simulink library "lib_dsphdlcontrol_v1"  (R2022a)
settings: Solver=ode45  StartTime=0.0  StopTime=10.0  RelTol=1e-3  EnableMultiTasking=on
undefined symbols (not defined in the file or in its folder): LIMIT, limit1, max1, min1, NumBits1, NumBits2, Slope1, Slope2, XMAX, XMIN
libraries: simulink x24, $bdroot x10, simulink_need_slupdate x5
settings Model: Creator=mbabst  LastModifiedBy=mbabst
settings SolverCC: AlgebraicLoopSolver=TrustRegion
settings DataIOCC: LimitDataPoints=on
settings OptimizationCC: LifeSpan=inf
settings DebuggingCC: UnconnectedInputMsg=warning  UnconnectedOutputMsg=warning  UnconnectedLineMsg=warning  AllowSymbolicDim=off  SFUnexpectedBacktrackingDiag=warning  SFNoUnconditionalDefaultTransitionDiag=warning  SFExecutionAtInitializationDiag=none  SFMachineParentedDataDiag=warning  ArithmeticOperatorsInVariantConditions=warning
settings SFSimCC: SimUseLocalCustomCode=off  CustomCodeUndefinedFunction=UseInterfaceOnly
settings RTWCC: RTWUseLocalCustomCode=off  DLArmComputeVersion=19.05
settings CodeAppCC: StateflowObjectComments=on
settings GRTTargetCC: TargetLangStandard=C89/C90 (ANSI)
settings ConfigComp: CovMetricSettings=dw  CovSaveCumulativeToWorkspaceVar=on  CovSaveSingleToWorkspaceVar=on  CovExternalEMLEnable=off

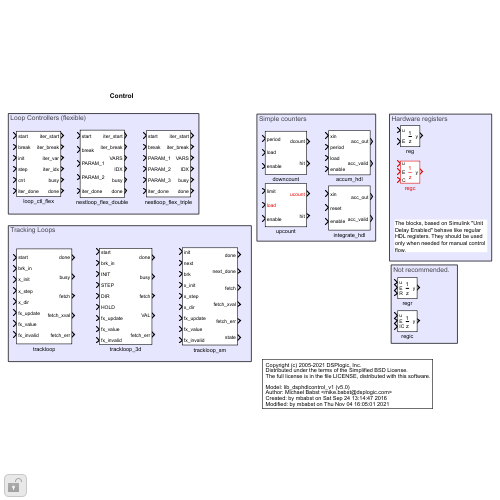
[thumbnail: Simulink's stored preview of the top-level diagram]
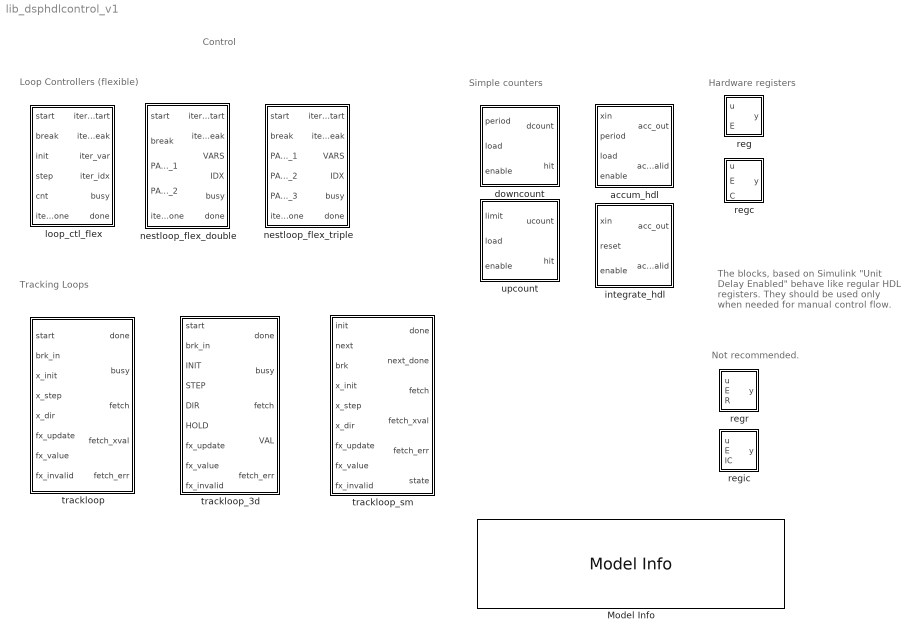
== system lib_dsphdlcontrol_v1 ==
  note: Not recommended.
  note: The blocks, based on Simulink "Unit Delay Enabled" behave like regular HDL registers. They should be used only when needed for manual control flow.
  note: Hardware registers
  note: Simple counters
  note: Tracking Loops
  note: Loop Controllers (flexible)
  note: Control
  Model Info : simulink/Model-Wide Utilities/Model Info  Frame=on  DisplayStringWithTags=|  HorizontalTextAlignment=Left  LeftAlignmentValue=0.02
      | Copyright (c) 2005-2021 DSPlogic, Inc.
      | Distributed under the terms of the Simplified BSD License.
      | The full license is in the file LICENSE, distributed with this software.
      | 
      | Model: %<ModelName> (v%<ModelVersion>)
      | Author: Michael Babst <mike.babst@dsplogic.com>
      | Created: by %<Creator> on %<Created>
      | Modified: by %<ModifiedBy> on %<LastModificationDate>
  accum_hdl : Subsystem  mask(HDL Accumulator){FreeRun=on}
      mask prompts: FreeRun "Free Running"
      mask help:
      | Free running or one-shot accumulator
      |
      | * Period should be set to the number of accumulations minus 1.
      | * Load initializes the accumulator and resets the current value to 0.
      | * Max number of accumulations is based upon width of period input.
      | * Output bit width is overflow safe, based on max number of accumulations
      mask init:
      | set_param([gcb '/downcount'],'FreeRun',FreeRun)
  downcount : Subsystem  mask(A simple down counter.){FreeRun=on}
      mask prompts: FreeRun "Free Running"
      mask help:
      | Period should be set to the desired period minus one.
      |
      | Hit will be asserted after Period enables.
      |
      | In free running mode, counter will roll over and begin again.  Otherwise, the counter operates in one-shot mode.
      |
      | The counter bit width is determined by the data type of the limit input.
      |
      | If load is never asserted, initial count will have one extra enable
  integrate_hdl : Subsystem  mask(HDL Accumulator){bit_growth=8}
      mask prompts: bit_growth "Accumulator Growth (bits)"
      mask help:
      | Free running accumulator
      |
      | * Load initializes the accumulator and resets the current value to 0.
      | * Max number of accumulations is based upon bit growth
  loop_ctl_flex : Subsystem  mask(Flexible Loop Controller){}
      mask help: This is loop controller intended to maximize control flexibility. It is not intended for tight loops where very low cycle overhead is desired. No attempt is made to pipeline execution of the iterated task.
      mask Help:
      | Author: Mike Babst <mike.babst@dsplogic.com>
      | Copyright (c) 2005-2016 DSPlogic, Inc.
  nestloop_flex_double : Subsystem  mask(Flexible Nested Loop (2-level)){}
      mask help: This is two level nested loop controller intended to maximize control flexibility. It is not intended for tight loops where very low cycle overhead is desired. No attempt is made to pipeline execution of the iterated task.
      mask Help:
      | Author: Mike Babst <mike.babst@dsplogic.com>
      | Copyright (c) 2005-2016 DSPlogic, Inc.
  nestloop_flex_triple : Subsystem  mask(Flexible Nested Loop (3-level)){}
      mask help: This is three level nested loop controller intended to maximize control flexibility. It is not intended for tight loops where very low cycle overhead is desired. No attempt is made to pipeline execution of the iterated task.
      mask Help:
      | Author: Mike Babst <mike.babst@dsplogic.com>
      | Copyright (c) 2005-2016 DSPlogic, Inc.
  reg : Subsystem  mask{vinit=0.0, tsamp=-1}
      mask prompts: vinit "Initial condition:"; tsamp "Sample time:"
      mask Display: dpoly(1,[1 0],'z')
  regc : Subsystem  mask{vinit=0.0, tsamp=-1}
      mask prompts: vinit "Initial condition:"; tsamp "Sample time:"
      mask Display: dpoly(1,[1 0],'z')
  regic : Subsystem  mask{tsamp=-1}
      mask prompts: tsamp "Sample time:"
      mask Display: dpoly(1,[1 0],'z')
  regr : Subsystem  mask{vinit=0.0, tsamp=-1}
      mask prompts: vinit "Initial condition:"; tsamp "Sample time:"
      mask Display: dpoly(1,[1 0],'z')
  trackloop : Subsystem  mask(Tracking Loop Controller){LIMIT=LIMIT, XMIN=XMIN, XMAX=XMAX}
      mask prompts: LIMIT "Limit X Range"; XMIN "Minimim allowed X"; XMAX "Maximum allowed X"
      mask help: This tracking loop performs a peak seach with a fixed step. If LIMIT is false, the range of X will be allowed to roll-over (positively or negatively) when the end of the fixed-point range is reached. If LIMIT is true, then XMIN and XMAX will be used to limit the range of X.
      mask Help:
      | Author: Mike Babst <mikebabst@gmail.com>
      | Copyright 2016 DSPlogic
  trackloop_3d : Subsystem  mask(Tracking Loop Controller){limit1=true, min1=0, max1=0.4, limit2=false, min2=0, max2=0, limit3=true, min3=0, max3=128}
      mask prompts: limit1 "LIMIT (true/false)"; min1 "Minimum value"; max1 "Maximum value"; limit2 "LIMIT (true/false)"; min2 "Minimum value"; max2 "Maximum value"; limit3 "Limit (true/false)"; min3 "Minimum value"; max3 "Maximum value"
      mask help: This tracking loop performs a peak seach with a fixed step. If LIMIT is false, the range of X will be allowed to roll-over (positively or negatively) when the end of the fixed-point range is reached. If LIMIT is true, then XMIN and XMAX will be used to limit the range of X.
      mask Help:
      | Author: Mike Babst <mikebabst@gmail.com>
      | Copyright 2016 DSPlogic
      mask DialogControl Container4 Prompt: Var1
      mask DialogControl Container7 Prompt: Var2
      mask DialogControl Container8 Prompt: Var3
  trackloop_sm : Subsystem  mask(Tracking Loop State Machine){LIMIT=limit1, XMIN=min1, XMAX=max1}
      mask prompts: LIMIT "Limit X Range"; XMIN "Minimum Allowed X"; XMAX "Maximum Allowed X"
      mask help: This tracking loop performs a peak seach with a fixed step. If LIMIT is false, the range of X will be allowed to roll-over (positively or negatively) when the end of the fixed-point range is reached. If LIMIT is true, then XMIN and XMAX will be used to limit the range of X.
      mask Help:
      | Author: Mike Babst <mikebabst@gmail.com>
      | Copyright 2016 DSPlogic
  upcount : Subsystem  mask(A simple down counter.){FreeRun=on}
      mask prompts: FreeRun "Free Running"
      mask help:
      | Period should be set to the desired period minus one.
      |
      | Hit will be asserted after Period enables.
      |
      | In free running mode, counter will roll over and begin again.  Otherwise, the counter operates in one-shot mode.
      |
      | The counter bit width is determined by the data type of the limit input.
      |
      | If load is never asserted, initial count will have one extra enable

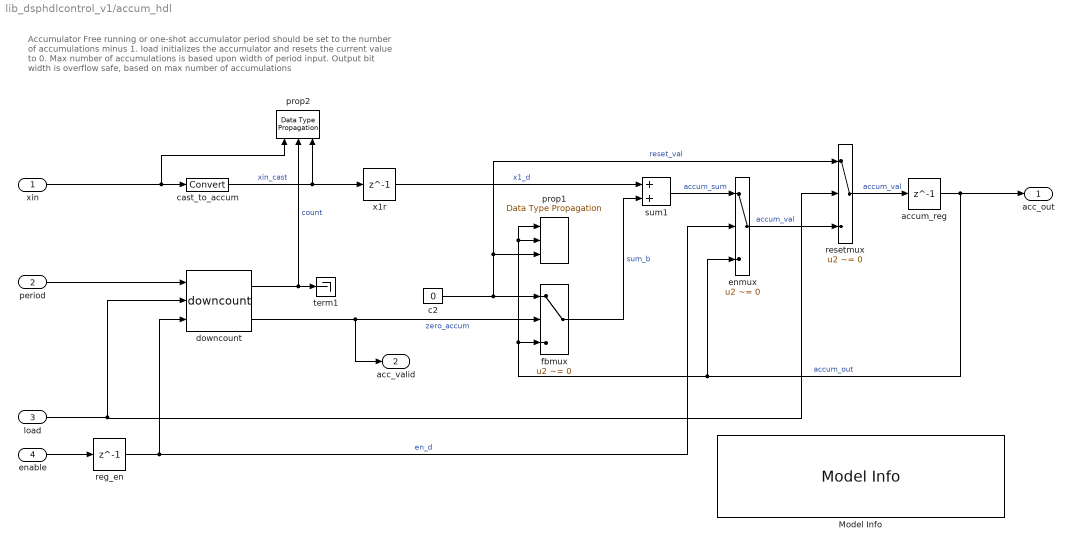
== system lib_dsphdlcontrol_v1/accum_hdl ==
  note: Accumulator
      | Free running or one-shot accumulator
      | period should be set to the number of accumulations minus 1.
      | load initializes the accumulator and resets the current value to 0.
      | Max number of accumulations is based upon width of period input.
      | Output bit width is overflow safe, based on max number of accumulations
  xin : Inport
  period : Inport  Port=2
  load : Inport  Port=3
  enable : Inport  Port=4
  Model Info : simulink/Model-Wide Utilities/Model Info  Frame=on  DisplayStringWithTags=|  HorizontalTextAlignment=Left  LeftAlignmentValue=0.02
      | Copyright (c) 2005-2021 DSPlogic, Inc.
      | Distributed under the terms of the Simplified BSD License.
      | The full license is in the file LICENSE, distributed with this software.
      | 
      | Model: %<ModelName> (v%<ModelVersion>)
      | Author: Michael Babst <mike.babst@dsplogic.com>
      | Created: by %<Creator> on %<Created>
      | Modified: by %<ModifiedBy> on %<LastModificationDate>
  accum_reg : Delay  DelayLength=1  InitialCondition=0
  c2 : Constant  Value=0  OutDataTypeStr=Inherit: Inherit via back propagation  SampleTime=-1
  cast_to_accum : DataTypeConversion  SaturateOnIntegerOverflow=off  RndMeth=Floor
  downcount : $bdroot/downcount  FreeRun=on
  enmux : Switch  Criteria=u2 ~= 0  SaturateOnIntegerOverflow=off  InputSameDT=off
  fbmux : Switch  Criteria=u2 ~= 0  SaturateOnIntegerOverflow=off  InputSameDT=off
  prop1 : simulink/Signal Attributes/Data Type Propagation  PropDataType=fixdt(1, 16)  IfRefDouble=double  IfRefSingle=single  IsSigned=IsSigned1 or IsSigned2  NumBitsBase=max([NumBits1 NumBits2])  NumBitsMult=1  NumBitsAdd=0  NumBitsAllowFinal=1:128  PropScaling=2^-10  ValuesUsedBestPrec=[5 -7]  SlopeBase=min([Slope1 Slope2])  SlopeMult=1  SlopeAdd=0  BiasBase=Bias1  BiasMult=1  BiasAdd=0
      settings: SourceProductBaseCode=SL
  prop2 : simulink/Signal Attributes/Data Type Propagation  PropDataType=fixdt(1, 16)  IfRefDouble=double  IfRefSingle=single  IsSigned=IsSigned1 or IsSigned2  NumBitsBase=NumBits1+NumBits2  NumBitsMult=1  NumBitsAdd=0  NumBitsAllowFinal=1:128  PropScaling=2^-10  ValuesUsedBestPrec=[5 -7]  SlopeBase=min([Slope1 Slope2])  SlopeMult=1  SlopeAdd=0  BiasBase=Bias1  BiasMult=1  BiasAdd=0
      settings: SourceProductBaseCode=SL
  reg_en : Delay  DelayLength=1  InitialCondition=0
  resetmux : Switch  Criteria=u2 ~= 0  SaturateOnIntegerOverflow=off  InputSameDT=off
  sum1 : Sum  OutDataTypeStr=Inherit: Same as first input
  term1 : Terminator
  x1r : Delay  DelayLength=1  InitialCondition=0
  acc_out : Outport
  acc_valid : Outport  Port=2
  wires:
  enmux/1 -> resetmux/3  "accum_val"
  xin/1 -> prop2/1, cast_to_accum/1
  resetmux/1 -> accum_reg/1  "accum_val"
  accum_reg/1 -> acc_out/1, fbmux/3, prop1/2, prop1/1, enmux/3  "accum_out"
  period/1 -> downcount/1
  load/1 -> downcount/2, resetmux/2
  cast_to_accum/1 -> prop2/3, x1r/1  "xin_cast"
  sum1/1 -> enmux/1  "accum_sum"
  c2/1 -> fbmux/1, prop1/3, resetmux/1  "reset_val"
  fbmux/1 -> sum1/2  "sum_b"
  downcount/2 -> fbmux/2, acc_valid/1  "zero_accum"
  x1r/1 -> sum1/1  "x1_d"
  enable/1 -> reg_en/1
  reg_en/1 -> downcount/3, enmux/2  "en_d"
  downcount/1 -> prop2/2, term1/1  "count"

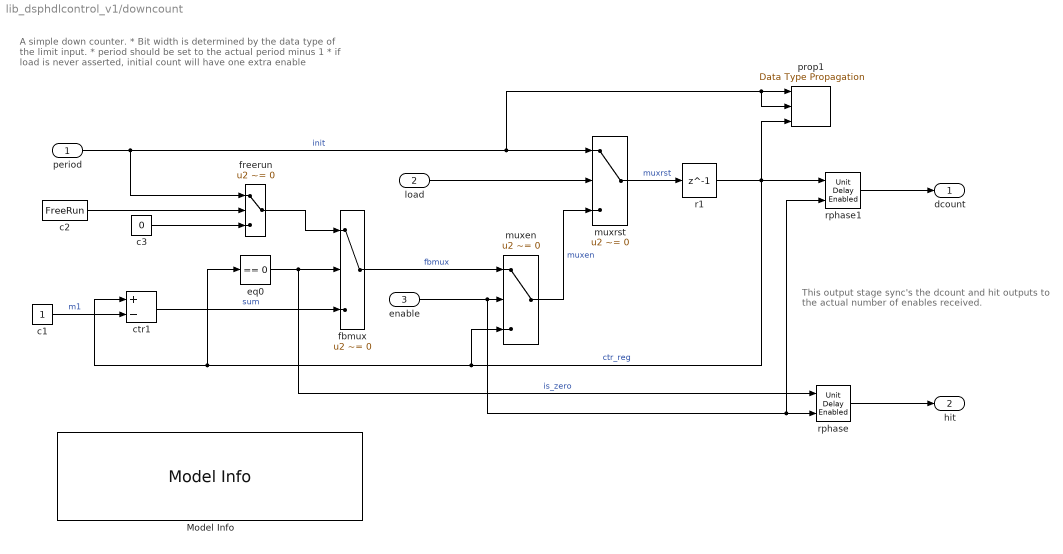
== system lib_dsphdlcontrol_v1/downcount ==
  note: A simple down counter.
      | * Bit width is determined by the data type of the limit input.
      | * period should be set to the actual period minus 1
      | * if load is never asserted, initial count will have one extra enable
  note: This output stage sync's the dcount and hit outputs
      | to the actual number of enables received.
  period : Inport
  load : Inport  Port=2  OutDataTypeStr=boolean
  enable : Inport  Port=3  OutDataTypeStr=boolean
  Model Info : simulink/Model-Wide Utilities/Model Info  Frame=on  DisplayStringWithTags=|  HorizontalTextAlignment=Left  LeftAlignmentValue=0.02
      | Copyright (c) 2005-2021 DSPlogic, Inc.
      | Distributed under the terms of the Simplified BSD License.
      | The full license is in the file LICENSE, distributed with this software.
      | 
      | Model: %<ModelName> (v%<ModelVersion>)
      | Author: Michael Babst <mike.babst@dsplogic.com>
      | Created: by %<Creator> on %<Created>
      | Modified: by %<ModifiedBy> on %<LastModificationDate>
  c1 : Constant  OutDataTypeStr=Inherit: Inherit via back propagation  SampleTime=-1
  c2 : Constant  Value=FreeRun  OutDataTypeStr=boolean  SampleTime=-1
  c3 : Constant  Value=0  OutDataTypeStr=Inherit: Inherit via back propagation  SampleTime=-1
  ctr1 : Sum  Inputs=+-  OutDataTypeStr=Inherit: Same as first input
  eq0 : simulink/Logic and Bit Operations/Compare To Constant  relop===  const=0  OutDataTypeStr=boolean
  fbmux : Switch  Criteria=u2 ~= 0  SaturateOnIntegerOverflow=off  InputSameDT=off
  freerun : Switch  Criteria=u2 ~= 0  SaturateOnIntegerOverflow=off  InputSameDT=off
  muxen : Switch  Criteria=u2 ~= 0  SaturateOnIntegerOverflow=off  InputSameDT=off
  muxrst : Switch  Criteria=u2 ~= 0  SaturateOnIntegerOverflow=off  InputSameDT=off
  prop1 : simulink/Signal Attributes/Data Type Propagation  PropDataType=fixdt(1, 16)  IfRefDouble=double  IfRefSingle=single  IsSigned=IsSigned1 or IsSigned2  NumBitsBase=max([NumBits1 NumBits2])  NumBitsMult=1  NumBitsAdd=0  NumBitsAllowFinal=1:128  PropScaling=2^-10  ValuesUsedBestPrec=[5 -7]  SlopeBase=min([Slope1 Slope2])  SlopeMult=1  SlopeAdd=0  BiasBase=Bias1  BiasMult=1  BiasAdd=0
      settings: SourceProductBaseCode=SL
  r1 : Delay  DelayLength=1  InitialCondition=0
  rphase : simulink_need_slupdate/Unit Delay Enabled  vinit=0.0  tsamp=-1
      settings: SourceProductBaseCode=SL
  rphase1 : simulink_need_slupdate/Unit Delay Enabled  vinit=0.0  tsamp=-1
      settings: SourceProductBaseCode=SL
  dcount : Outport
  hit : Outport  Port=2
  wires:
  enable/1 -> muxen/2, rphase/2, rphase1/2
  rphase1/1 -> dcount/1
  rphase/1 -> hit/1
  c3/1 -> freerun/3
  c2/1 -> freerun/2
  freerun/1 -> fbmux/1
  period/1 -> prop1/2, prop1/1, muxrst/1, freerun/1  "init"
  muxrst/1 -> r1/1  "muxrst"
  muxen/1 -> muxrst/3  "muxen"
  r1/1 -> prop1/3, muxen/3, eq0/1, ctr1/1, rphase1/1  "ctr_reg"
  load/1 -> muxrst/2
  fbmux/1 -> muxen/1  "fbmux"
  c1/1 -> ctr1/2  "m1"
  eq0/1 -> fbmux/2, rphase/1  "is_zero"
  ctr1/1 -> fbmux/3  "sum"

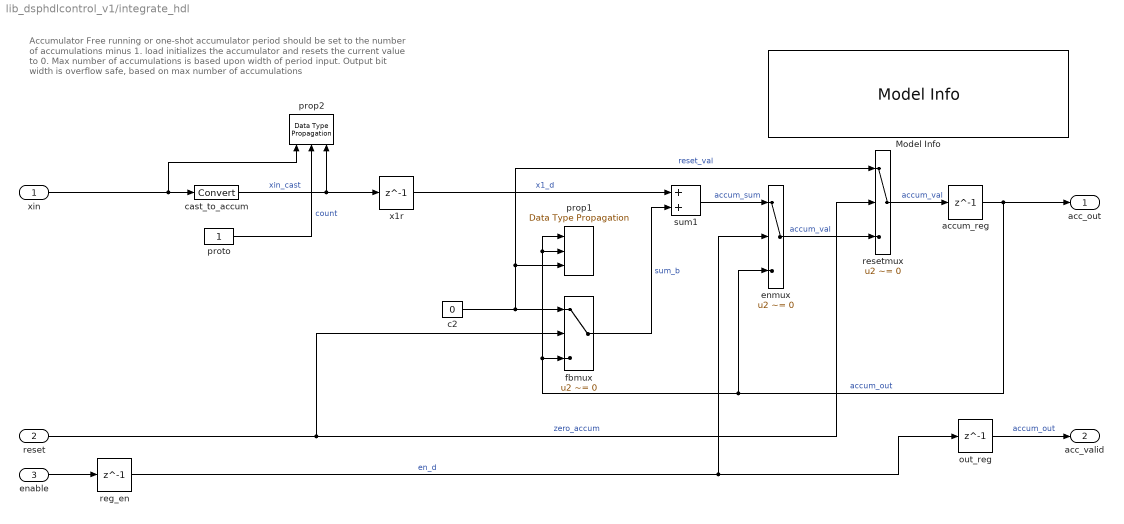
== system lib_dsphdlcontrol_v1/integrate_hdl ==
  note: Accumulator
      | Free running or one-shot accumulator
      | period should be set to the number of accumulations minus 1.
      | load initializes the accumulator and resets the current value to 0.
      | Max number of accumulations is based upon width of period input.
      | Output bit width is overflow safe, based on max number of accumulations
  xin : Inport
  reset : Inport  Port=2
  enable : Inport  Port=3
  Model Info : simulink/Model-Wide Utilities/Model Info  Frame=on  DisplayStringWithTags=|  HorizontalTextAlignment=Left  LeftAlignmentValue=0.02
      | Copyright (c) 2005-2021 DSPlogic, Inc.
      | Distributed under the terms of the Simplified BSD License.
      | The full license is in the file LICENSE, distributed with this software.
      | 
      | Model: %<ModelName> (v%<ModelVersion>)
      | Author: Michael Babst <mike.babst@dsplogic.com>
      | Created: by %<Creator> on %<Created>
      | Modified: by %<ModifiedBy> on %<LastModificationDate>
  accum_reg : Delay  DelayLength=1  InitialCondition=0
  c2 : Constant  Value=0  OutDataTypeStr=Inherit: Inherit via back propagation  SampleTime=-1
  cast_to_accum : DataTypeConversion  SaturateOnIntegerOverflow=off  RndMeth=Floor
  enmux : Switch  Criteria=u2 ~= 0  SaturateOnIntegerOverflow=off  InputSameDT=off
  fbmux : Switch  Criteria=u2 ~= 0  SaturateOnIntegerOverflow=off  InputSameDT=off
  out_reg : Delay  DelayLength=1  InitialCondition=0
  prop1 : simulink/Signal Attributes/Data Type Propagation  PropDataType=fixdt(1, 16)  IfRefDouble=double  IfRefSingle=single  IsSigned=IsSigned1 or IsSigned2  NumBitsBase=max([NumBits1 NumBits2])  NumBitsMult=1  NumBitsAdd=0  NumBitsAllowFinal=1:128  PropScaling=2^-10  ValuesUsedBestPrec=[5 -7]  SlopeBase=min([Slope1 Slope2])  SlopeMult=1  SlopeAdd=0  BiasBase=Bias1  BiasMult=1  BiasAdd=0
      settings: SourceProductBaseCode=SL
  prop2 : simulink/Signal Attributes/Data Type Propagation  PropDataType=fixdt(1, 16)  IfRefDouble=double  IfRefSingle=single  IsSigned=IsSigned1 or IsSigned2  NumBitsBase=NumBits1+NumBits2  NumBitsMult=1  NumBitsAdd=0  NumBitsAllowFinal=1:128  PropScaling=2^-10  ValuesUsedBestPrec=[5 -7]  SlopeBase=min([Slope1 Slope2])  SlopeMult=1  SlopeAdd=0  BiasBase=Bias1  BiasMult=1  BiasAdd=0
      settings: SourceProductBaseCode=SL
  proto : Constant  OutDataTypeStr=fixdt(0,bit_growth,0)  SampleTime=-1
  reg_en : Delay  DelayLength=1  InitialCondition=0
  resetmux : Switch  Criteria=u2 ~= 0  SaturateOnIntegerOverflow=off  InputSameDT=off
  sum1 : Sum  OutDataTypeStr=Inherit: Same as first input
  x1r : Delay  DelayLength=1  InitialCondition=0
  acc_out : Outport
  acc_valid : Outport  Port=2
  wires:
  out_reg/1 -> acc_valid/1  "accum_out"
  proto/1 -> prop2/2  "count"
  reg_en/1 -> enmux/2, out_reg/1  "en_d"
  enable/1 -> reg_en/1
  x1r/1 -> sum1/1  "x1_d"
  reset/1 -> fbmux/2, resetmux/2  "zero_accum"
  fbmux/1 -> sum1/2  "sum_b"
  c2/1 -> resetmux/1, prop1/3, fbmux/1  "reset_val"
  sum1/1 -> enmux/1  "accum_sum"
  cast_to_accum/1 -> x1r/1, prop2/3  "xin_cast"
  accum_reg/1 -> enmux/3, prop1/1, prop1/2, fbmux/3, acc_out/1  "accum_out"
  resetmux/1 -> accum_reg/1  "accum_val"
  xin/1 -> cast_to_accum/1, prop2/1
  enmux/1 -> resetmux/3  "accum_val"

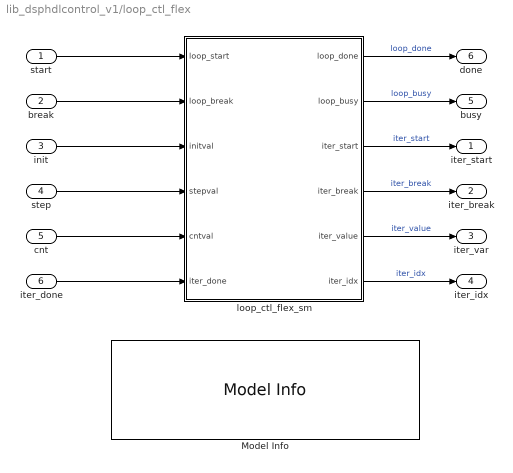
== system lib_dsphdlcontrol_v1/loop_ctl_flex ==
  start : Inport
  break : Inport  Port=2
  init : Inport  Port=3
  step : Inport  Port=4
  cnt : Inport  Port=5
  iter_done : Inport  Port=6
  Model Info : simulink/Model-Wide Utilities/Model Info  Frame=on  DisplayStringWithTags=|  HorizontalTextAlignment=Left  LeftAlignmentValue=0.02
      | Copyright (c) 2005-2021 DSPlogic, Inc.
      | Distributed under the terms of the Simplified BSD License.
      | The full license is in the file LICENSE, distributed with this software.
      | 
      | Model: %<ModelName> (v%<ModelVersion>)
      | Author: Michael Babst <mike.babst@dsplogic.com>
      | Created: by %<Creator> on %<Created>
      | Modified: by %<ModifiedBy> on %<LastModificationDate>
  loop_ctl_flex_sm : MATLAB Function  TreatAsAtomicUnit=on
  iter_start : Outport
  iter_break : Outport  Port=2
  iter_var : Outport  Port=3
  iter_idx : Outport  Port=4
  busy : Outport  Port=5
  done : Outport  Port=6
  wires:
  loop_ctl_flex_sm/4(iter_break) -> iter_break/1  "iter_break"
  break/1 -> loop_ctl_flex_sm/2(loop_break)
  init/1 -> loop_ctl_flex_sm/3(initval)
  start/1 -> loop_ctl_flex_sm/1(loop_start)
  step/1 -> loop_ctl_flex_sm/4(stepval)
  cnt/1 -> loop_ctl_flex_sm/5(cntval)
  iter_done/1 -> loop_ctl_flex_sm/6(iter_done)
  loop_ctl_flex_sm/1(loop_done) -> done/1  "loop_done"
  loop_ctl_flex_sm/2(loop_busy) -> busy/1  "loop_busy"
  loop_ctl_flex_sm/3(iter_start) -> iter_start/1  "iter_start"
  loop_ctl_flex_sm/5(iter_value) -> iter_var/1  "iter_value"
  loop_ctl_flex_sm/6(iter_idx) -> iter_idx/1  "iter_idx"

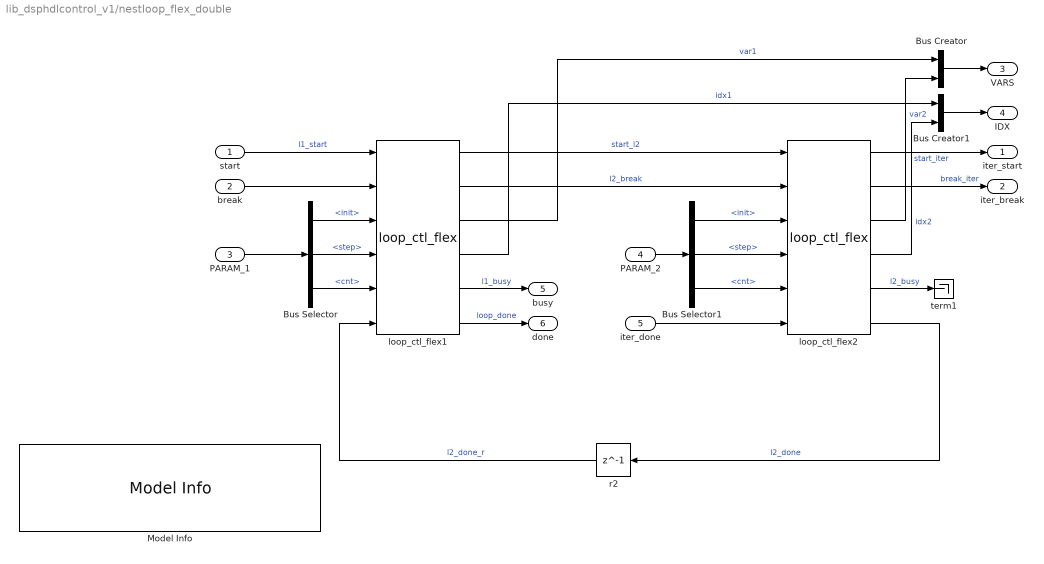
== system lib_dsphdlcontrol_v1/nestloop_flex_double ==
  start : Inport
  break : Inport  Port=2
  PARAM_1 : Inport  Port=3
  PARAM_2 : Inport  Port=4
  iter_done : Inport  Port=5
  Bus Creator : BusCreator  Inputs=2
  Bus Creator1 : BusCreator  Inputs=2
  Bus Selector : BusSelector  OutputSignals=init,step,cnt
  Bus Selector1 : BusSelector  OutputSignals=init,step,cnt
  Model Info : simulink/Model-Wide Utilities/Model Info  Frame=on  DisplayStringWithTags=|  HorizontalTextAlignment=Left  LeftAlignmentValue=0.02
      | Copyright (c) 2005-2021 DSPlogic, Inc.
      | Distributed under the terms of the Simplified BSD License.
      | The full license is in the file LICENSE, distributed with this software.
      | 
      | Model: %<ModelName> (v%<ModelVersion>)
      | Author: Michael Babst <mike.babst@dsplogic.com>
      | Created: by %<Creator> on %<Created>
      | Modified: by %<ModifiedBy> on %<LastModificationDate>
  loop_ctl_flex1 : $bdroot/loop_ctl_flex
  loop_ctl_flex2 : $bdroot/loop_ctl_flex
  r2 : Delay  DelayLength=1  InitialCondition=0
  term1 : Terminator
  iter_start : Outport
  iter_break : Outport  Port=2
  VARS : Outport  Port=3
  IDX : Outport  Port=4
  busy : Outport  Port=5
  done : Outport  Port=6
  wires:
  loop_ctl_flex2/6 -> r2/1  "l2_done"
  Bus Creator1/1 -> IDX/1
  loop_ctl_flex2/4 -> Bus Creator1/2  "idx2"
  loop_ctl_flex1/4 -> Bus Creator1/1  "idx1"
  Bus Creator/1 -> VARS/1
  loop_ctl_flex2/3 -> Bus Creator/2  "var2"
  loop_ctl_flex1/3 -> Bus Creator/1  "var1"
  loop_ctl_flex2/5 -> term1/1  "l2_busy"
  loop_ctl_flex2/2 -> iter_break/1  "break_iter"
  loop_ctl_flex1/6 -> done/1  "loop_done"
  PARAM_2/1 -> Bus Selector1/1
  loop_ctl_flex1/5 -> busy/1  "l1_busy"
  iter_done/1 -> loop_ctl_flex2/6
  Bus Selector1/3 -> loop_ctl_flex2/5  "<cnt>"
  Bus Selector1/2 -> loop_ctl_flex2/4  "<step>"
  Bus Selector1/1 -> loop_ctl_flex2/3  "<init>"
  Bus Selector/3 -> loop_ctl_flex1/5  "<cnt>"
  Bus Selector/2 -> loop_ctl_flex1/4  "<step>"
  Bus Selector/1 -> loop_ctl_flex1/3  "<init>"
  PARAM_1/1 -> Bus Selector/1
  r2/1 -> loop_ctl_flex1/6  "l2_done_r"
  loop_ctl_flex1/1 -> loop_ctl_flex2/1  "start_l2"
  start/1 -> loop_ctl_flex1/1  "l1_start"
  break/1 -> loop_ctl_flex1/2
  loop_ctl_flex1/2 -> loop_ctl_flex2/2  "l2_break"
  loop_ctl_flex2/1 -> iter_start/1  "start_iter"

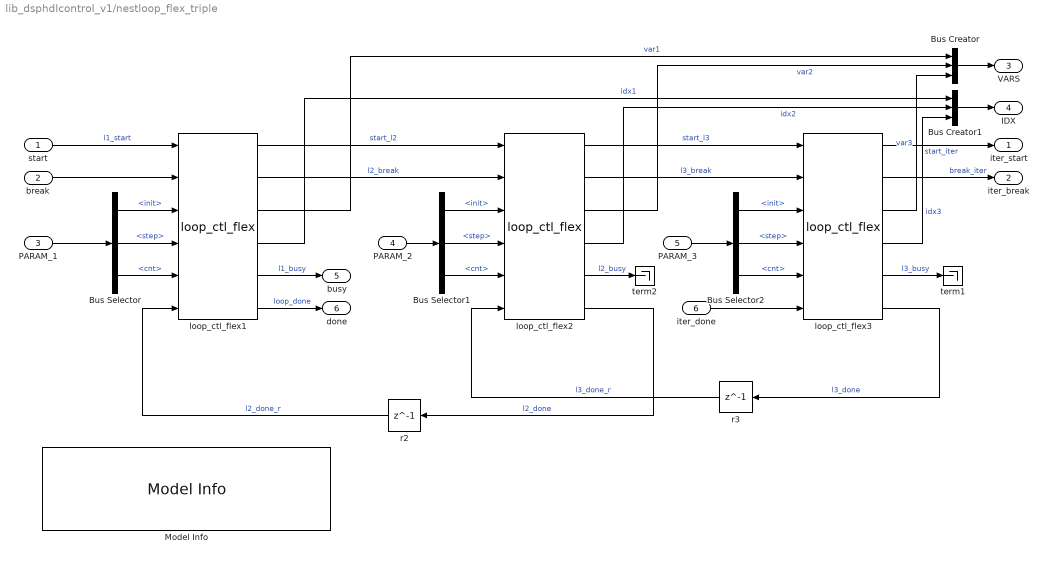
== system lib_dsphdlcontrol_v1/nestloop_flex_triple ==
  start : Inport
  break : Inport  Port=2
  PARAM_1 : Inport  Port=3
  PARAM_2 : Inport  Port=4
  PARAM_3 : Inport  Port=5
  iter_done : Inport  Port=6
  Bus Creator : BusCreator  Inputs=3
  Bus Creator1 : BusCreator  Inputs=3
  Bus Selector : BusSelector  OutputSignals=init,step,cnt
  Bus Selector1 : BusSelector  OutputSignals=init,step,cnt
  Bus Selector2 : BusSelector  OutputSignals=init,step,cnt
  Model Info : simulink/Model-Wide Utilities/Model Info  Frame=on  DisplayStringWithTags=|  HorizontalTextAlignment=Left  LeftAlignmentValue=0.02
      | Copyright (c) 2005-2021 DSPlogic, Inc.
      | Distributed under the terms of the Simplified BSD License.
      | The full license is in the file LICENSE, distributed with this software.
      | 
      | Model: %<ModelName> (v%<ModelVersion>)
      | Author: Michael Babst <mike.babst@dsplogic.com>
      | Created: by %<Creator> on %<Created>
      | Modified: by %<ModifiedBy> on %<LastModificationDate>
  loop_ctl_flex1 : $bdroot/loop_ctl_flex
  loop_ctl_flex2 : $bdroot/loop_ctl_flex
  loop_ctl_flex3 : $bdroot/loop_ctl_flex
  r2 : Delay  DelayLength=1  InitialCondition=0
  r3 : Delay  DelayLength=1  InitialCondition=0
  term1 : Terminator
  term2 : Terminator
  iter_start : Outport
  iter_break : Outport  Port=2
  VARS : Outport  Port=3
  IDX : Outport  Port=4
  busy : Outport  Port=5
  done : Outport  Port=6
  wires:
  loop_ctl_flex3/1 -> iter_start/1  "start_iter"
  loop_ctl_flex2/2 -> loop_ctl_flex3/2  "l3_break"
  loop_ctl_flex1/2 -> loop_ctl_flex2/2  "l2_break"
  break/1 -> loop_ctl_flex1/2
  start/1 -> loop_ctl_flex1/1  "l1_start"
  loop_ctl_flex1/1 -> loop_ctl_flex2/1  "start_l2"
  loop_ctl_flex2/6 -> r2/1  "l2_done"
  r2/1 -> loop_ctl_flex1/6  "l2_done_r"
  loop_ctl_flex2/1 -> loop_ctl_flex3/1  "start_l3"
  loop_ctl_flex3/6 -> r3/1  "l3_done"
  r3/1 -> loop_ctl_flex2/6  "l3_done_r"
  PARAM_1/1 -> Bus Selector/1
  Bus Selector/1 -> loop_ctl_flex1/3  "<init>"
  Bus Selector/2 -> loop_ctl_flex1/4  "<step>"
  Bus Selector/3 -> loop_ctl_flex1/5  "<cnt>"
  Bus Selector1/1 -> loop_ctl_flex2/3  "<init>"
  Bus Selector1/2 -> loop_ctl_flex2/4  "<step>"
  Bus Selector1/3 -> loop_ctl_flex2/5  "<cnt>"
  Bus Selector2/1 -> loop_ctl_flex3/3  "<init>"
  Bus Selector2/2 -> loop_ctl_flex3/4  "<step>"
  Bus Selector2/3 -> loop_ctl_flex3/5  "<cnt>"
  iter_done/1 -> loop_ctl_flex3/6
  loop_ctl_flex1/5 -> busy/1  "l1_busy"
  PARAM_2/1 -> Bus Selector1/1
  PARAM_3/1 -> Bus Selector2/1
  loop_ctl_flex1/6 -> done/1  "loop_done"
  loop_ctl_flex3/2 -> iter_break/1  "break_iter"
  loop_ctl_flex3/5 -> term1/1  "l3_busy"
  loop_ctl_flex2/5 -> term2/1  "l2_busy"
  loop_ctl_flex1/3 -> Bus Creator/1  "var1"
  loop_ctl_flex2/3 -> Bus Creator/2  "var2"
  loop_ctl_flex3/3 -> Bus Creator/3  "var3"
  Bus Creator/1 -> VARS/1
  loop_ctl_flex1/4 -> Bus Creator1/1  "idx1"
  loop_ctl_flex2/4 -> Bus Creator1/2  "idx2"
  loop_ctl_flex3/4 -> Bus Creator1/3  "idx3"
  Bus Creator1/1 -> IDX/1

== system lib_dsphdlcontrol_v1/reg ==
  u : Inport
  E : Inport  Port=2
  Delay : Delay  DelayLength=1  InitialCondition=vinit  SampleTime=tsamp
  Enable : Switch  Criteria=u2 ~= 0  OutDataTypeStr=Inherit: Inherit via back propagation  ZeroCross=off  SaturateOnIntegerOverflow=off  InputSameDT=off
  FixPt Data Type Duplicate1 : DataTypeDuplicate  DisableCoverage=on  NumInputPorts=3
  Model Info : simulink/Model-Wide Utilities/Model Info  Frame=on  DisplayStringWithTags=|  HorizontalTextAlignment=Left  LeftAlignmentValue=0.02
      | Copyright (c) 2005-2021 DSPlogic, Inc.
      | Distributed under the terms of the Simplified BSD License.
      | The full license is in the file LICENSE, distributed with this software.
      | 
      | Model: %<ModelName> (v%<ModelVersion>)
      | Author: Michael Babst <mike.babst@dsplogic.com>
      | Created: by %<Creator> on %<Created>
      | Modified: by %<ModifiedBy> on %<LastModificationDate>
  y : Outport
  wires:
  Delay/1 -> FixPt Data Type Duplicate1/1, Enable/3, y/1  "y"
  Enable/1 -> FixPt Data Type Duplicate1/2, Delay/1  "ynext"
  u/1 -> Enable/1, FixPt Data Type Duplicate1/3
  E/1 -> Enable/2

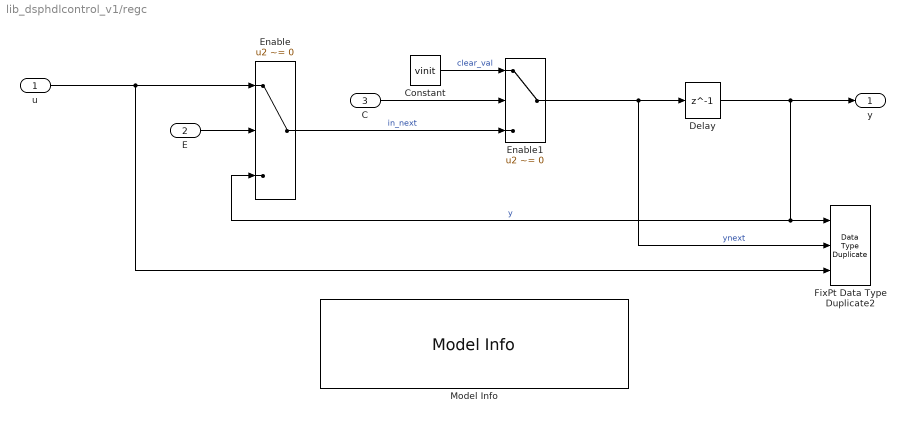
== system lib_dsphdlcontrol_v1/regc ==
  u : Inport
  E : Inport  Port=2
  C : Inport  Port=3
  Constant : Constant  Value=vinit  OutDataTypeStr=Inherit: Inherit via back propagation  SampleTime=tsamp
  Delay : Delay  DelayLength=1  InitialCondition=vinit  SampleTime=tsamp
  Enable : Switch  Criteria=u2 ~= 0  OutDataTypeStr=Inherit: Inherit via back propagation  ZeroCross=off  SaturateOnIntegerOverflow=off  InputSameDT=off
  Enable1 : Switch  Criteria=u2 ~= 0  OutDataTypeStr=Inherit: Inherit via back propagation  ZeroCross=off  SaturateOnIntegerOverflow=off  InputSameDT=off
  FixPt Data Type Duplicate2 : DataTypeDuplicate  DisableCoverage=on  NumInputPorts=3
  Model Info : simulink/Model-Wide Utilities/Model Info  Frame=on  DisplayStringWithTags=|  HorizontalTextAlignment=Left  LeftAlignmentValue=0.02
      | Copyright (c) 2005-2021 DSPlogic, Inc.
      | Distributed under the terms of the Simplified BSD License.
      | The full license is in the file LICENSE, distributed with this software.
      | 
      | Model: %<ModelName> (v%<ModelVersion>)
      | Author: Michael Babst <mike.babst@dsplogic.com>
      | Created: by %<Creator> on %<Created>
      | Modified: by %<ModifiedBy> on %<LastModificationDate>
  y : Outport
  wires:
  Enable/1 -> Enable1/3  "in_next"
  u/1 -> Enable/1, FixPt Data Type Duplicate2/3
  C/1 -> Enable1/2
  Constant/1 -> Enable1/1  "clear_val"
  Enable1/1 -> FixPt Data Type Duplicate2/2, Delay/1  "ynext"
  E/1 -> Enable/2
  Delay/1 -> y/1, FixPt Data Type Duplicate2/1, Enable/3  "y"

== system lib_dsphdlcontrol_v1/regic ==
  note: Initial Value
  note: Enable
  u : Inport
  E : Inport  Port=2
  IC : Inport  Port=3
  Enable : Switch  Criteria=u2 ~= 0  OutDataTypeStr=Inherit: Inherit via back propagation  ZeroCross=off  SaturateOnIntegerOverflow=off  InputSameDT=off
  FixPt Data Type Duplicate1 : DataTypeDuplicate  DisableCoverage=on  NumInputPorts=4
  Model Info : simulink/Model-Wide Utilities/Model Info  Frame=on  DisplayStringWithTags=|  HorizontalTextAlignment=Left  LeftAlignmentValue=0.02
      | Copyright (c) 2005-2021 DSPlogic, Inc.
      | Distributed under the terms of the Simplified BSD License.
      | The full license is in the file LICENSE, distributed with this software.
      | 
      | Model: %<ModelName> (v%<ModelVersion>)
      | Author: Michael Babst <mike.babst@dsplogic.com>
      | Created: by %<Creator> on %<Created>
      | Modified: by %<ModifiedBy> on %<LastModificationDate>
  State Control : StateControl  DisableCoverage=on
  Unit Delay External IC : simulink_need_slupdate/Unit Delay External IC  tsamp=tsamp
      settings: SourceProductBaseCode=SL
  y : Outport
  wires:
  Unit Delay External IC/1 -> FixPt Data Type Duplicate1/1, Enable/3, y/1
  Enable/1 -> Unit Delay External IC/1, FixPt Data Type Duplicate1/2  "Xnew"
  u/1 -> Enable/1, FixPt Data Type Duplicate1/4
  IC/1 -> Unit Delay External IC/2, FixPt Data Type Duplicate1/3
  E/1 -> Enable/2

== system lib_dsphdlcontrol_v1/regr ==
  note: Enable
  u : Inport
  E : Inport  Port=2
  R : Inport  Port=3
  Delay : Delay  DelayLength=1  InitialCondition=vinit  ExternalReset=Level  SampleTime=tsamp
      settings: InputPortMap=u0,r5
  Enable : Switch  Criteria=u2 ~= 0  OutDataTypeStr=Inherit: Inherit via back propagation  ZeroCross=off  SaturateOnIntegerOverflow=off  InputSameDT=off
  FixPt Data Type Duplicate2 : DataTypeDuplicate  DisableCoverage=on  NumInputPorts=3
  Model Info : simulink/Model-Wide Utilities/Model Info  Frame=on  DisplayStringWithTags=|  HorizontalTextAlignment=Left  LeftAlignmentValue=0.02
      | Copyright (c) 2005-2021 DSPlogic, Inc.
      | Distributed under the terms of the Simplified BSD License.
      | The full license is in the file LICENSE, distributed with this software.
      | 
      | Model: %<ModelName> (v%<ModelVersion>)
      | Author: Michael Babst <mike.babst@dsplogic.com>
      | Created: by %<Creator> on %<Created>
      | Modified: by %<ModifiedBy> on %<LastModificationDate>
  y : Outport
  wires:
  R/1 -> Delay/2
  E/1 -> Enable/2
  u/1 -> Enable/1, FixPt Data Type Duplicate2/3
  Enable/1 -> Delay/1, FixPt Data Type Duplicate2/2  "xnew"
  Delay/1 -> y/1, FixPt Data Type Duplicate2/1, Enable/3

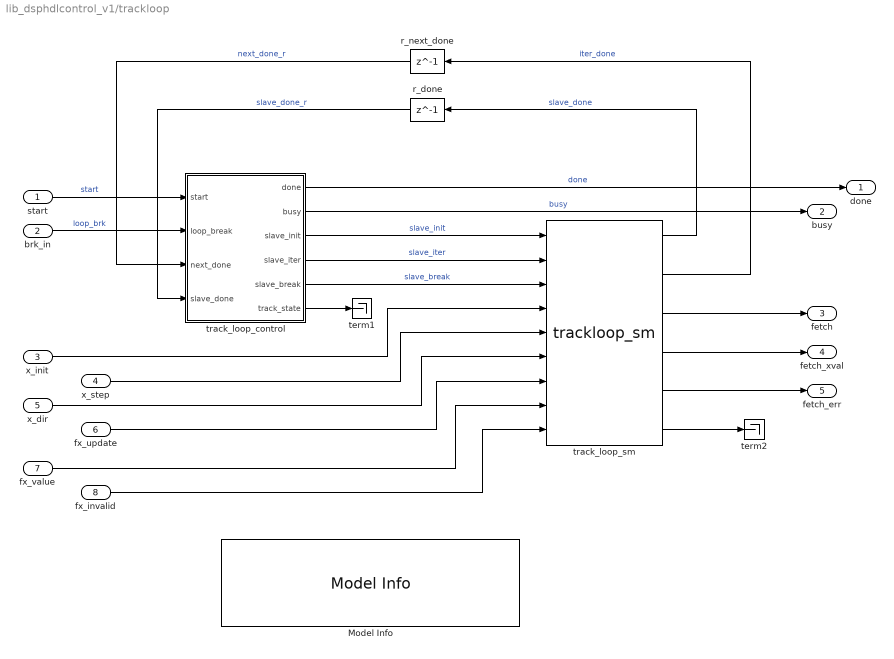
== system lib_dsphdlcontrol_v1/trackloop ==
  start : Inport
  brk_in : Inport  Port=2
  x_init : Inport  Port=3
  x_step : Inport  Port=4
  x_dir : Inport  Port=5
  fx_update : Inport  Port=6
  fx_value : Inport  Port=7
  fx_invalid : Inport  Port=8
  Model Info : simulink/Model-Wide Utilities/Model Info  Frame=on  DisplayStringWithTags=|  HorizontalTextAlignment=Left  LeftAlignmentValue=0.02
      | Copyright (c) 2005-2021 DSPlogic, Inc.
      | Distributed under the terms of the Simplified BSD License.
      | The full license is in the file LICENSE, distributed with this software.
      | 
      | Model: %<ModelName> (v%<ModelVersion>)
      | Author: Michael Babst <mike.babst@dsplogic.com>
      | Created: by %<Creator> on %<Created>
      | Modified: by %<ModifiedBy> on %<LastModificationDate>
  r_done : Delay  DelayLength=1  InitialCondition=0
  r_next_done : Delay  DelayLength=1  InitialCondition=0
  term1 : Terminator
  term2 : Terminator
  track_loop_control : MATLAB Function  TreatAsAtomicUnit=on
  track_loop_sm : $bdroot/trackloop_sm  LIMIT=LIMIT  XMIN=XMIN  XMAX=XMAX
  done : Outport
  busy : Outport  Port=2
  fetch : Outport  Port=3
  fetch_xval : Outport  Port=4
  fetch_err : Outport  Port=5
  wires:
  track_loop_control/6(track_state) -> term1/1
  track_loop_control/2(busy) -> busy/1  "busy"
  x_step/1 -> track_loop_sm/5
  x_init/1 -> track_loop_sm/4
  x_dir/1 -> track_loop_sm/6
  r_next_done/1 -> track_loop_control/3(next_done)  "next_done_r"
  track_loop_sm/1 -> r_done/1  "slave_done"
  track_loop_sm/2 -> r_next_done/1  "iter_done"
  fx_update/1 -> track_loop_sm/7
  fx_value/1 -> track_loop_sm/8
  fx_invalid/1 -> track_loop_sm/9
  track_loop_sm/3 -> fetch/1
  track_loop_sm/4 -> fetch_xval/1
  track_loop_sm/5 -> fetch_err/1
  track_loop_sm/6 -> term2/1
  track_loop_control/1(done) -> done/1  "done"
  track_loop_control/5(slave_break) -> track_loop_sm/3  "slave_break"
  track_loop_control/4(slave_iter) -> track_loop_sm/2  "slave_iter"
  track_loop_control/3(slave_init) -> track_loop_sm/1  "slave_init"
  start/1 -> track_loop_control/1(start)  "start"
  r_done/1 -> track_loop_control/4(slave_done)  "slave_done_r"
  brk_in/1 -> track_loop_control/2(loop_break)  "loop_brk"

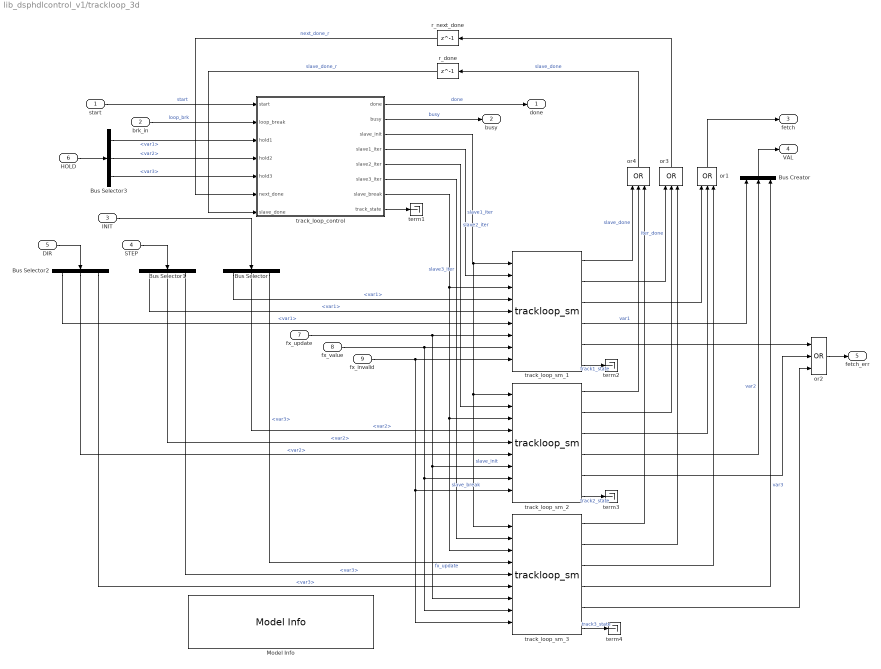
== system lib_dsphdlcontrol_v1/trackloop_3d ==
  start : Inport
  brk_in : Inport  Port=2
  INIT : Inport  Port=3
  STEP : Inport  Port=4
  DIR : Inport  Port=5
  HOLD : Inport  Port=6
  fx_update : Inport  Port=7
  fx_value : Inport  Port=8
  fx_invalid : Inport  Port=9
  Bus Creator : BusCreator  Inputs=3
  Bus Selector{,1..3} (4 alike) : BusSelector  OutputSignals=var1,var2,var3
  Model Info : simulink/Model-Wide Utilities/Model Info  Frame=on  DisplayStringWithTags=|  HorizontalTextAlignment=Left  LeftAlignmentValue=0.02
      | Copyright (c) 2005-2021 DSPlogic, Inc.
      | Distributed under the terms of the Simplified BSD License.
      | The full license is in the file LICENSE, distributed with this software.
      | 
      | Model: %<ModelName> (v%<ModelVersion>)
      | Author: Michael Babst <mike.babst@dsplogic.com>
      | Created: by %<Creator> on %<Created>
      | Modified: by %<ModifiedBy> on %<LastModificationDate>
  or{1..4} (4 alike) : Logic  Operator=OR  Inputs=3  IconShape=distinctive  AllPortsSameDT=off  OutDataTypeStr=boolean
  r_done : Delay  DelayLength=1  InitialCondition=0
  r_next_done : Delay  DelayLength=1  InitialCondition=0
  term{1..4} (4 alike) : Terminator
  track_loop_control : MATLAB Function  TreatAsAtomicUnit=on
  track_loop_sm_1 : $bdroot/trackloop_sm  LIMIT=limit1  XMIN=min1  XMAX=max1
  track_loop_sm_2 : $bdroot/trackloop_sm  LIMIT=limit2  XMIN=min2  XMAX=max2
  track_loop_sm_3 : $bdroot/trackloop_sm  LIMIT=limit3  XMIN=min3  XMAX=max3
  done : Outport
  busy : Outport  Port=2
  fetch : Outport  Port=3
  VAL : Outport  Port=4
  fetch_err : Outport  Port=5
  wires:
  Bus Selector3/3 -> track_loop_control/5(hold3)  "<var3>"
  Bus Selector3/2 -> track_loop_control/4(hold2)  "<var2>"
  Bus Selector3/1 -> track_loop_control/3(hold1)  "<var1>"
  HOLD/1 -> Bus Selector3/1
  track_loop_control/6(slave3_iter) -> track_loop_sm_3/2  "slave3_iter"
  track_loop_control/5(slave2_iter) -> track_loop_sm_2/2  "slave2_iter"
  Bus Selector2/3 -> track_loop_sm_3/6  "<var3>"
  Bus Selector2/2 -> track_loop_sm_2/6  "<var2>"
  Bus Selector2/1 -> track_loop_sm_1/6  "<var1>"
  DIR/1 -> Bus Selector2/1
  Bus Selector1/3 -> track_loop_sm_3/5  "<var3>"
  Bus Selector1/2 -> track_loop_sm_2/5  "<var2>"
  Bus Selector1/1 -> track_loop_sm_1/5  "<var1>"
  STEP/1 -> Bus Selector1/1
  Bus Selector/3 -> track_loop_sm_3/4  "<var3>"
  Bus Selector/2 -> track_loop_sm_2/4  "<var2>"
  Bus Selector/1 -> track_loop_sm_1/4  "<var1>"
  track_loop_sm_3/1 -> or4/3
  track_loop_sm_2/1 -> or4/2
  track_loop_sm_1/1 -> or4/1  "slave_done"
  or3/1 -> r_next_done/1
  track_loop_sm_3/2 -> or3/3
  track_loop_sm_2/2 -> or3/2
  or2/1 -> fetch_err/1
  track_loop_sm_3/5 -> or2/3
  track_loop_sm_2/5 -> or2/2
  track_loop_sm_1/5 -> or2/1
  Bus Creator/1 -> VAL/1
  track_loop_sm_3/6 -> term4/1  "track3_state"
  track_loop_sm_2/6 -> term3/1  "track2_state"
  track_loop_sm_3/4 -> Bus Creator/3  "var3"
  track_loop_sm_2/4 -> Bus Creator/2  "var2"
  track_loop_sm_1/4 -> Bus Creator/1  "var1"
  track_loop_sm_3/3 -> or1/3
  track_loop_sm_2/3 -> or1/2
  track_loop_sm_1/3 -> or1/1
  or1/1 -> fetch/1
  track_loop_control/8(track_state) -> term1/1
  track_loop_control/2(busy) -> busy/1  "busy"
  INIT/1 -> Bus Selector/1
  r_next_done/1 -> track_loop_control/6(next_done)  "next_done_r"
  or4/1 -> r_done/1  "slave_done"
  track_loop_sm_1/2 -> or3/1  "iter_done"
  fx_update/1 -> track_loop_sm_1/7, track_loop_sm_2/7, track_loop_sm_3/7  "fx_update"
  fx_value/1 -> track_loop_sm_1/8, track_loop_sm_2/8, track_loop_sm_3/8
  fx_invalid/1 -> track_loop_sm_1/9, track_loop_sm_2/9, track_loop_sm_3/9
  track_loop_sm_1/6 -> term2/1  "track1_state"
  track_loop_control/1(done) -> done/1  "done"
  track_loop_control/7(slave_break) -> track_loop_sm_1/3, track_loop_sm_2/3, track_loop_sm_3/3  "slave_break"
  track_loop_control/4(slave1_iter) -> track_loop_sm_1/2  "slave1_iter"
  track_loop_control/3(slave_init) -> track_loop_sm_1/1, track_loop_sm_2/1, track_loop_sm_3/1  "slave_init"
  start/1 -> track_loop_control/1(start)  "start"
  r_done/1 -> track_loop_control/7(slave_done)  "slave_done_r"
  brk_in/1 -> track_loop_control/2(loop_break)  "loop_brk"

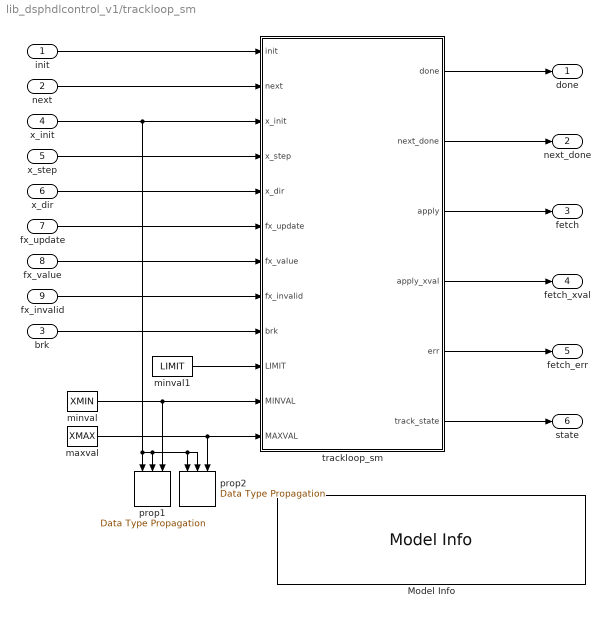
== system lib_dsphdlcontrol_v1/trackloop_sm ==
  init : Inport
  next : Inport  Port=2
  brk : Inport  Port=3
  x_init : Inport  Port=4
  x_step : Inport  Port=5
  x_dir : Inport  Port=6
  fx_update : Inport  Port=7
  fx_value : Inport  Port=8
  fx_invalid : Inport  Port=9
  Model Info : simulink/Model-Wide Utilities/Model Info  Frame=on  DisplayStringWithTags=|  HorizontalTextAlignment=Left  LeftAlignmentValue=0.02
      | Copyright (c) 2005-2021 DSPlogic, Inc.
      | Distributed under the terms of the Simplified BSD License.
      | The full license is in the file LICENSE, distributed with this software.
      | 
      | Model: %<ModelName> (v%<ModelVersion>)
      | Author: Michael Babst <mike.babst@dsplogic.com>
      | Created: by %<Creator> on %<Created>
      | Modified: by %<ModifiedBy> on %<LastModificationDate>
  maxval : Constant  Value=XMAX  OutDataTypeStr=Inherit: Inherit via back propagation  SampleTime=-1
  minval : Constant  Value=XMIN  OutDataTypeStr=Inherit: Inherit via back propagation  SampleTime=-1
  minval1 : Constant  Value=LIMIT  OutDataTypeStr=boolean  SampleTime=-1
  prop1 : simulink/Signal Attributes/Data Type Propagation  PropDataType=fixdt(1, 16)  IfRefDouble=double  IfRefSingle=single  IsSigned=IsSigned1 or IsSigned2  NumBitsBase=max([NumBits1 NumBits2])  NumBitsMult=1  NumBitsAdd=0  NumBitsAllowFinal=1:128  PropScaling=2^-10  ValuesUsedBestPrec=[5 -7]  SlopeBase=min([Slope1 Slope2])  SlopeMult=1  SlopeAdd=0  BiasBase=Bias1  BiasMult=1  BiasAdd=0
      settings: SourceProductBaseCode=SL
  prop2 : simulink/Signal Attributes/Data Type Propagation  PropDataType=fixdt(1, 16)  IfRefDouble=double  IfRefSingle=single  IsSigned=IsSigned1 or IsSigned2  NumBitsBase=max([NumBits1 NumBits2])  NumBitsMult=1  NumBitsAdd=0  NumBitsAllowFinal=1:128  PropScaling=2^-10  ValuesUsedBestPrec=[5 -7]  SlopeBase=min([Slope1 Slope2])  SlopeMult=1  SlopeAdd=0  BiasBase=Bias1  BiasMult=1  BiasAdd=0
      settings: SourceProductBaseCode=SL
  trackloop_sm : MATLAB Function  TreatAsAtomicUnit=on
  done : Outport
  next_done : Outport  Port=2
  fetch : Outport  Port=3
  fetch_xval : Outport  Port=4
  fetch_err : Outport  Port=5
  state : Outport  Port=6
  wires:
  minval1/1 -> trackloop_sm/10(LIMIT)
  trackloop_sm/5(err) -> fetch_err/1
  fx_invalid/1 -> trackloop_sm/8(fx_invalid)
  trackloop_sm/2(next_done) -> next_done/1
  trackloop_sm/6(track_state) -> state/1
  minval/1 -> trackloop_sm/11(MINVAL), prop1/3
  x_dir/1 -> trackloop_sm/5(x_dir)
  trackloop_sm/1(done) -> done/1
  fx_value/1 -> trackloop_sm/7(fx_value)
  brk/1 -> trackloop_sm/9(brk)
  x_step/1 -> trackloop_sm/4(x_step)
  next/1 -> trackloop_sm/2(next)
  trackloop_sm/4(apply_xval) -> fetch_xval/1
  fx_update/1 -> trackloop_sm/6(fx_update)
  init/1 -> trackloop_sm/1(init)
  x_init/1 -> prop2/2, prop2/1, prop1/2, prop1/1, trackloop_sm/3(x_init)
  trackloop_sm/3(apply) -> fetch/1
  maxval/1 -> trackloop_sm/12(MAXVAL), prop2/3

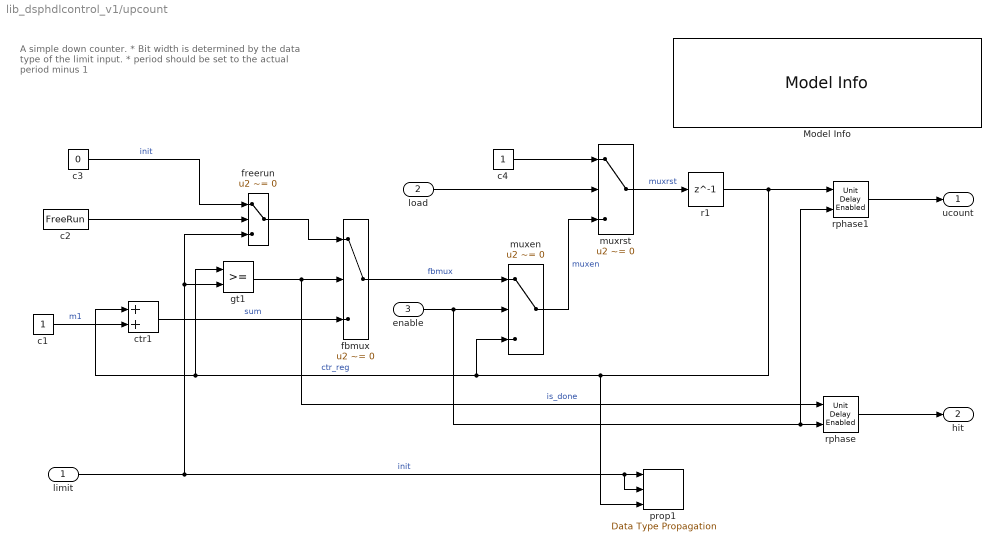
== system lib_dsphdlcontrol_v1/upcount ==
  note: A simple down counter.
      | * Bit width is determined by the data type of the limit input.
      | * period should be set to the actual period minus 1
  limit : Inport
  load : Inport  Port=2  OutDataTypeStr=boolean
  enable : Inport  Port=3  OutDataTypeStr=boolean
  Model Info : simulink/Model-Wide Utilities/Model Info  Frame=on  DisplayStringWithTags=|  HorizontalTextAlignment=Left  LeftAlignmentValue=0.02
      | Copyright (c) 2005-2021 DSPlogic, Inc.
      | Distributed under the terms of the Simplified BSD License.
      | The full license is in the file LICENSE, distributed with this software.
      | 
      | Model: %<ModelName> (v%<ModelVersion>)
      | Author: Michael Babst <mike.babst@dsplogic.com>
      | Created: by %<Creator> on %<Created>
      | Modified: by %<ModifiedBy> on %<LastModificationDate>
  c1 : Constant  OutDataTypeStr=Inherit: Inherit via back propagation  SampleTime=-1
  c2 : Constant  Value=FreeRun  OutDataTypeStr=boolean  SampleTime=-1
  c3 : Constant  Value=0  OutDataTypeStr=Inherit: Inherit via back propagation  SampleTime=-1
  c4 : Constant  OutDataTypeStr=Inherit: Inherit via back propagation  SampleTime=-1
  ctr1 : Sum  OutDataTypeStr=Inherit: Same as first input
  fbmux : Switch  Criteria=u2 ~= 0  SaturateOnIntegerOverflow=off  InputSameDT=off
  freerun : Switch  Criteria=u2 ~= 0  SaturateOnIntegerOverflow=off  InputSameDT=off
  gt1 : RelationalOperator  OutDataTypeStr=boolean  InputSameDT=off
  muxen : Switch  Criteria=u2 ~= 0  SaturateOnIntegerOverflow=off  InputSameDT=off
  muxrst : Switch  Criteria=u2 ~= 0  SaturateOnIntegerOverflow=off  InputSameDT=off
  prop1 : simulink/Signal Attributes/Data Type Propagation  PropDataType=fixdt(1, 16)  IfRefDouble=double  IfRefSingle=single  IsSigned=IsSigned1 or IsSigned2  NumBitsBase=max([NumBits1 NumBits2])  NumBitsMult=1  NumBitsAdd=0  NumBitsAllowFinal=1:128  PropScaling=2^-10  ValuesUsedBestPrec=[5 -7]  SlopeBase=min([Slope1 Slope2])  SlopeMult=1  SlopeAdd=0  BiasBase=Bias1  BiasMult=1  BiasAdd=0
      settings: SourceProductBaseCode=SL
  r1 : Delay  DelayLength=1  InitialCondition=0
  rphase : simulink_need_slupdate/Unit Delay Enabled  vinit=0.0  tsamp=-1
      settings: SourceProductBaseCode=SL
  rphase1 : simulink_need_slupdate/Unit Delay Enabled  vinit=0.0  tsamp=-1
      settings: SourceProductBaseCode=SL
  ucount : Outport
  hit : Outport  Port=2
  wires:
  c4/1 -> muxrst/1
  enable/1 -> muxen/2, rphase/2, rphase1/2
  rphase1/1 -> ucount/1
  rphase/1 -> hit/1
  c2/1 -> freerun/2
  freerun/1 -> fbmux/1
  c3/1 -> freerun/1  "init"
  muxrst/1 -> r1/1  "muxrst"
  muxen/1 -> muxrst/3  "muxen"
  r1/1 -> rphase1/1, prop1/3, muxen/3, gt1/1, ctr1/1  "ctr_reg"
  load/1 -> muxrst/2
  fbmux/1 -> muxen/1  "fbmux"
  c1/1 -> ctr1/2  "m1"
  gt1/1 -> fbmux/2, rphase/1  "is_done"
  ctr1/1 -> fbmux/3  "sum"
  limit/1 -> freerun/3, gt1/2, prop1/1, prop1/2  "init"

== matlab function lib_dsphdlcontrol_v1/trackloop_sm/trackloop_sm ==
  settings: fimath=hdlMath()
  data: init input; done output; next input; x_init input; x_step input; x_dir input; fx_update input boolean; fx_value input; fx_invalid input; brk input; LIMIT input; MINVAL input; MAXVAL input; next_done output; apply output; apply_xval output; err output; track_state output
function [ done,...
           next_done,...
           apply,...
           apply_xval,...
           err,...
           track_state]...
  = fcn( ...
           init,...
           next,...
           x_init,...
           x_step,...
           x_dir,...
           fx_update,... 
           fx_value,...
           fx_invalid,...
           brk,...
           LIMIT,...
           MINVAL,...
           MAXVAL...
)%#codegen
         [ done,...
           next_done,...
           apply,...
           apply_xval,...
           err,...
           track_state]...
  = trackloop_sm( ...
           init,...
           next,...
           x_init,...
           x_step,...
           x_dir,...
           fx_update,... 
           fx_value,...
           fx_invalid,...
           brk,...
           LIMIT,...
           MINVAL,...
           MAXVAL...
);%#codegen

== matlab function lib_dsphdlcontrol_v1/loop_ctl_flex/loop_ctl_flex_sm ==
  data: loop_done output boolean; loop_busy output; loop_start input boolean; loop_break input; initval input; stepval input; cntval input; iter_start output boolean; iter_break output; iter_done input boolean; iter_value output; iter_idx output
function [ loop_done, loop_busy, iter_start, iter_break, iter_value, iter_idx ] = loop_ctl_flex( ...
           loop_start, loop_break, initval, stepval, cntval, iter_done ...   
)%#codegen
         [ loop_done, loop_busy, iter_start, iter_break, iter_value, iter_idx ] = loop_ctl_flex_sm( ...
           loop_start, loop_break, initval, stepval, cntval, iter_done...   
);

== matlab function lib_dsphdlcontrol_v1/trackloop/track_loop_control ==
  settings: fimath=hdlMath()
  data: start input boolean; loop_break input boolean; done output boolean; busy output boolean; next_done input boolean; slave_init output boolean; slave_iter output boolean; slave_break output boolean; track_state output; slave_done input boolean
function [ done,...
           busy,...
           slave_init,...
           slave_iter,...
           slave_break,...
           track_state]...
  = track_loop_control( ...
           start,...
           loop_break,...
           next_done,...
           slave_done...
)%#codegen
% TRACK_LOOP_CONTROL
%   
% Description:
%   A top level loop controller that handles control flow for
%   the peak finder state machine.
% 
% Author: mike babst <mike.babst@dsplogic.com>
% Copyright 2016 DSPlogic

%% Define Constants
[state, Wstate] = getStates();     % Main states


%% Define Registers
persistent state_r;
persistent init_r;
persistent done_r;
persistent slave_iter_r;
persistent slave_break_r;
persistent busy_r;
persistent loop_broken_r;
if isempty(state_r)
    state_r  = hdlu(state.idle, Wstate);
    init_r = false;
    done_r = false;
    slave_iter_r = false;
    slave_break_r = false;
    busy_r = false;
    loop_broken_r = false;
end

%% Assign outputs
track_state = state_r;
slave_init = init_r;
done = done_r;
slave_iter = slave_iter_r;
slave_break = slave_break_r;
busy = busy_r;

    %% Capture break input and pass through
    if loop_break
        loop_broken_r = true;
    end
    


    %% Main state machine
    % Default values
    done_r   = false;
    init_r   = false;
    slave_iter_r = false;
    slave_break_r  = false;
    
    switch state_r
        
        case state.idle
            
            loop_broken_r = false;
            busy_r = false;
            
            if start
                state_r = hdlu(state.init, Wstate);
                init_r = true;
                busy_r = true;
            end
                
        case state.init
            % Wait for slave_init to complete
            if next_done
                if ~loop_broken_r
                    %Prepare for slave_iter
                    slave_iter_r = true;
                    state_r = hdlu(state.slave_iter, Wstate);
                else
                    state_r = hdlu(state.broken, Wstate);
                end                    
            end
            
        case state.slave_iter
            % Wait for slave to complete
            if next_done
                if ~loop_broken_r
                    %Prepare for slave_iter
                    slave_iter_r = true;
                    state_r = hdlu(state.slave_iter, Wstate);
                else
                    state_r = hdlu(state.broken, Wstate);
                end
                
            end

        case state.broken
            %% Wait for slave to break
            slave_break_r = true;
            if slave_done
                state_r = hdlu(state.idle, Wstate);
                busy_r = false;
                done_r = true;               
                slave_break_r = true;
            end                

            
        otherwise
            state_r = hdlu(state.idle, Wstate);
            busy_r = false;
            done_r = true;               

    end
    
end



function [state, Wstate] = getStates()
    % State bit width
    Wstate = 4;
    state.idle         = 0;
    state.init         = 1;
    state.slave_iter   = 2;
    state.error        = 3;
    state.broken       = 4;
end

== matlab function lib_dsphdlcontrol_v1/trackloop_3d/track_loop_control ==
  settings: fimath=hdlMath()
  data: start input boolean; loop_break input boolean; hold1 input; hold2 input; hold3 input; done output boolean; busy output boolean; next_done input boolean; slave_init output boolean; slave1_iter output boolean; slave2_iter output; slave3_iter output; slave_break output boolean; track_state output; slave_done input boolean
function [ done,...
           busy,...
           slave_init,...
           slave1_iter,...
           slave2_iter,...
           slave3_iter,...
           slave_break,...
           track_state]...
  = trackloop_3d_ctl( ...
           start,...
           loop_break,...
           hold1,...
           hold2,...
           hold3,...
           next_done,...
           slave_done...
)%#codegen
         [ done,...
           busy,...
           slave_init,...
           slave1_iter,...
           slave2_iter,...
           slave3_iter,...
           slave_break,...
           track_state]...
  = trackloop_3d_ctl( ...
           start,...
           loop_break,...
           hold1,...
           hold2,...
           hold3,...
           next_done,...
           slave_done...
);%#codegen
